simulink model "quadcopter_model_MAIN"  (R2022b)
settings: Solver=FixedStepAuto  StartTime=0.0  StopTime=inf  FixedStep=0.002  RelTol=1e-3
values from neighbouring files (symbols this model uses):
  altToPrsBias = 101270.95    [load_model_parameters.m]
  altToPrsGain = 12.0173    [load_model_parameters.m]
  D = zeros(size(C,1), size(B,2))    [integral_state_feedback.m]    (also in output_feedback.m)
  inverse_mixer_matrix = [1  1  1  1 ... (first row only)    [load_model_parameters.m]
  ms2_to_mg = (1/9.80665)*1000    (= 101.971621298)    [load_model_parameters.m]
  ms_to_cms = 100    [load_model_parameters.m]
  SampleTime = 0.002    [load_model_parameters.m]
undefined symbols (not defined in the file or in its folder): Payload
libraries: uavmavlinklib x11, simulink x3, px4MAVLinkBridgelib x2, robotcorelib x2, sharedtransform x1, sensorinslib x1, mspsensorlib x1
settings Model: ExtModeTrigDuration=10  Creator=paolo  LastModifiedBy=paolo

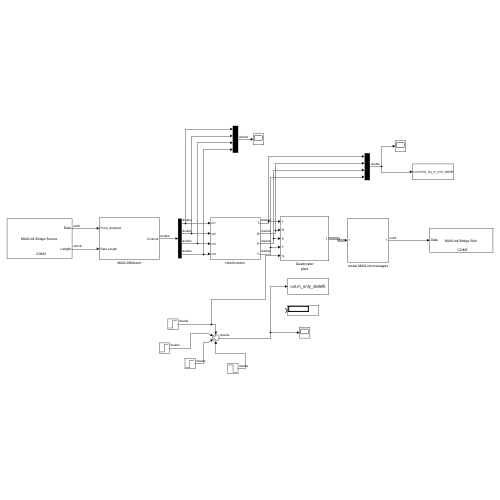
[thumbnail: Simulink's stored preview of the top-level diagram]
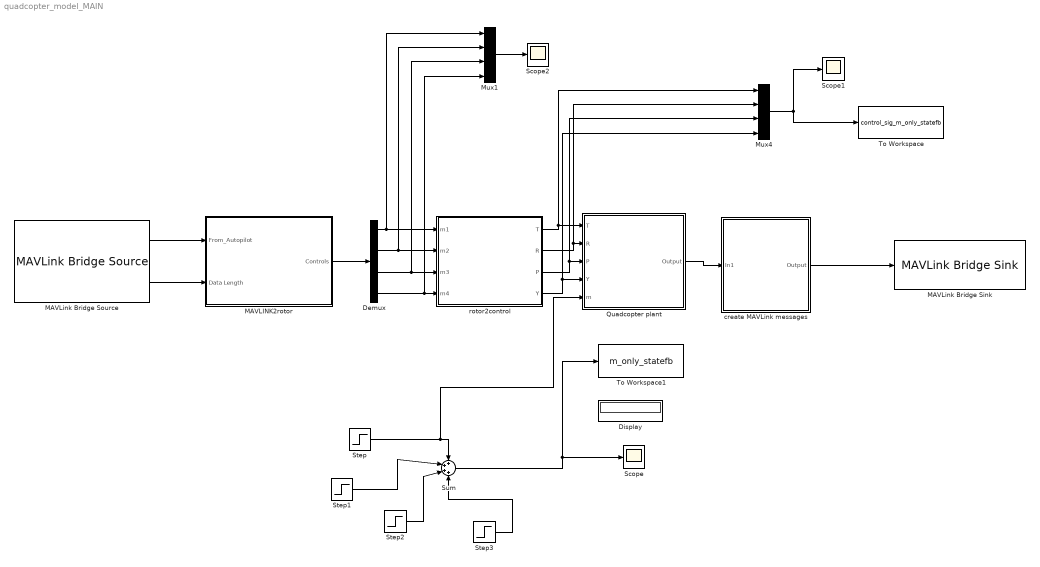
== system quadcopter_model_MAIN ==
  Demux : Demux
  Display : Display
  MAVLINK2rotor : Subsystem
  MAVLink Bridge Sink : px4MAVLinkBridgelib/MAVLink Bridge Sink  PixhawkSerialPorttemp=Specify manually  PixhawkSerialPortManually=COM3  FieldTable={ 'UDP', '127.0.0.1', '14550' }
  MAVLink Bridge Source : px4MAVLinkBridgelib/MAVLink Bridge Source  PixhawkSerialPorttemp=Specify manually  PixhawkSerialPortManually=COM3  dataLength=1024  FieldTable={ 'UDP', '127.0.0.1', '14550' }  SampleTime=SampleTime
  Mux1 : Mux
  Mux4 : Mux
  Quadcopter plant : Subsystem
  Scope : Scope
  Scope1 : Scope
  Scope2 : Scope
  Step : Step  Time=0  After=1.2  SampleTime=0
  Step1 : Step  Time=20  After=1.2  SampleTime=0
  Step2 : Step  Time=40  After=1.2  SampleTime=0
  Step3 : Step  Time=70  After=-2.4  SampleTime=0
  Sum : Sum  Inputs=++++
  To Workspace : ToWorkspace  VariableName=control_sig_m_only_statefb  SampleTime=-1
  To Workspace1 : ToWorkspace  VariableName=m_only_statefb  SampleTime=-1
  create MAVLink messages : Subsystem
  "rotor2control " : Subsystem
  wires:
  Demux/2 -> Mux1/2, "rotor2control "/2(m2)
  Demux/1 -> Mux1/1, "rotor2control "/1(m1)
  Demux/3 -> Mux1/3, "rotor2control "/3(m3)
  Demux/4 -> Mux1/4, "rotor2control "/4(m4)
  Quadcopter plant/1(Output) -> create MAVLink messages/1(In1)
  MAVLink Bridge Source/1 -> MAVLINK2rotor/1(From_Autopilot)
  MAVLink Bridge Source/2 -> MAVLINK2rotor/2(Data Length)
  MAVLINK2rotor/1(Controls) -> Demux/1
  "rotor2control "/3(P) -> Mux4/3, Quadcopter plant/3(P)
  "rotor2control "/4(Y) -> Mux4/4, Quadcopter plant/4(Y)
  "rotor2control "/1(T) -> Mux4/1, Quadcopter plant/1(T)
  "rotor2control "/2(R) -> Mux4/2, Quadcopter plant/2(R)
  Mux4/1 -> To Workspace/1, Scope1/1
  Mux1/1 -> Scope2/1
  Sum/1 -> To Workspace1/1, Scope/1
  Step/1 -> Quadcopter plant/5(m), Sum/1
  Step1/1 -> Sum/2
  Step2/1 -> Sum/3
  Step3/1 -> Sum/4
  create MAVLink messages/1(Output) -> MAVLink Bridge Sink/1

== system quadcopter_model_MAIN/MAVLINK2rotor ==
  From_Autopilot : Inport
  Data Length : Inport  Port=2
  Enabled Subsystem1 : Subsystem  TreatAsAtomicUnit=on
  "Input Signal " : Subsystem
  Controls : Outport
  wires:
  Enabled Subsystem1/1(Controls) -> Controls/1
  Data Length/1 -> "Input Signal "/2(Data Length)
  "Input Signal "/1(Signal) -> Enabled Subsystem1/1(byteStreamInput)
  From_Autopilot/1 -> "Input Signal "/1(From_Autopilot)

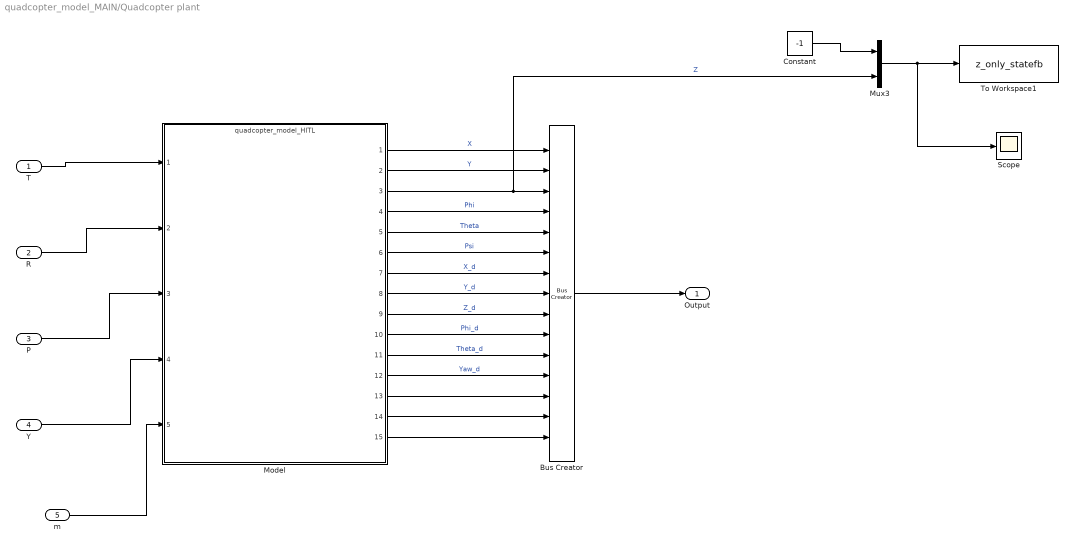
== system quadcopter_model_MAIN/Quadcopter plant ==
  T : Inport
  R : Inport  Port=2
  P : Inport  Port=3
  Y : Inport  Port=4
  m : Inport  Port=5
  Bus Creator : BusCreator  Inputs=15
  Constant : Constant  Value=-1
  Model : ModelReference  ModelNameDialog=quadcopter_model_HITL.slx  SimulationMode=Normal  ModelReferenceVersion=1.131
  Mux3 : Mux  Inputs=2
  Scope : Scope
  To Workspace1 : ToWorkspace  VariableName=z_only_statefb  SampleTime=-1
  Output : Outport
  wires:
  Bus Creator/1 -> Output/1
  R/1 -> Model/2
  T/1 -> Model/1
  P/1 -> Model/3
  Y/1 -> Model/4
  Model/1 -> Bus Creator/1  "X"
  Model/2 -> Bus Creator/2  "Y"
  Model/3 -> Mux3/2, Bus Creator/3  "Z"
  Model/4 -> Bus Creator/4  "Phi"
  Model/5 -> Bus Creator/5  "Theta"
  Model/6 -> Bus Creator/6  "Psi"
  Model/7 -> Bus Creator/7  "X_d"
  Model/8 -> Bus Creator/8  "Y_d"
  Model/9 -> Bus Creator/9  "Z_d"
  Model/10 -> Bus Creator/10  "Phi_d"
  Model/11 -> Bus Creator/11  "Theta_d"
  Model/12 -> Bus Creator/12  "Yaw_d"
  Model/13 -> Bus Creator/13
  Model/14 -> Bus Creator/14
  Model/15 -> Bus Creator/15
  Mux3/1 -> Scope/1, To Workspace1/1
  m/1 -> Model/5
  Constant/1 -> Mux3/1

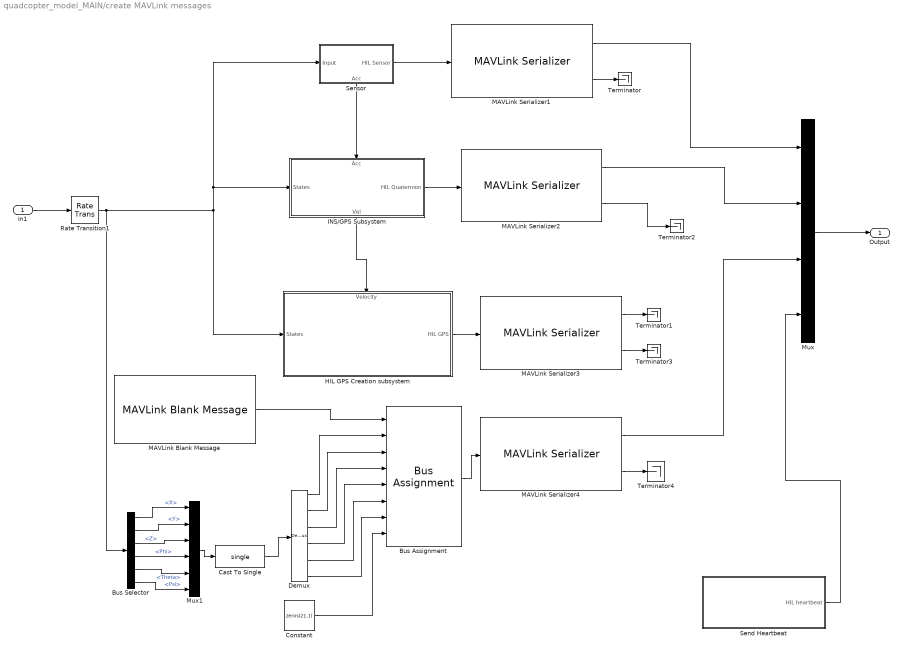
== system quadcopter_model_MAIN/create MAVLink messages ==
  In1 : Inport
  Bus Assignment : BusAssignment  AssignedSignals=Payload.x,Payload.y,Payload.z,Payload.roll,Payload.pitch,Payload.yaw,Payload.covariance
  Bus Selector : BusSelector  OutputSignals=X,Y,Z,Phi,Theta,Psi
  Cast To Single : DataTypeConversion  OutDataTypeStr=single  SaturateOnIntegerOverflow=off  RndMeth=Floor
  Constant : Constant  Value=zeros(21,1)  OutDataTypeStr=single
  Demux : Demux  Outputs=6
  HIL GPS Creation subsystem : Subsystem
      settings: PortSchema="{\"entries\":[{\"content\":{\"sides\":[{\"content\":{\"connectorIds\":[\"In1\"]},\"type\":\"ConnectorPlacement.EquallySpacedRectSide\",\"uuid\":\"f4444677-f205-4bd8-9e95-5e6060697dc4\"},{\"content\":{\"connectorIds\":[\"Out1\"],\"side\":\"RIGHT\"},\"type\":\"ConnectorPlacement.EquallySpacedRectSide\",\"uuid\":\"c948a3e0-826b-4d7b-9e4f-6e3881854d5a\"},{\"content\":{\"connectorIds\":[\"In2\"],\"side\":\"TOP\"},\"type\":\"ConnectorPlacement.EquallySpacedRectSide\",\"uuid\":\"82cf0daf-0b59-4b3c-ab0e-258a514f37ad\"},{\"content\":{\"connectorIds\":[],\"side\":\"HIDDEN\"},\"type\":\"ConnectorPlacement.EquallySpacedRectSide\",\"uuid\":\"a794f320-9150-4c05-acf0-96079b0d3066\"}]},\"type\":\"ConnectorPlacement.EquallySpacedConnector\",\"uuid\":\"8d0915ff-9064-46da-be4f-31886e994f25\"}],\"packageUris\":[\"http://schema.mathworks.com/mf0/Connector/R2020b\"],\"version\":\"1.0\"}"
  INS/GPS Subsystem : Subsystem
      settings: PortSchema="{\"entries\":[{\"content\":{\"sides\":[{\"content\":{\"connectorIds\":[\"In1\"]},\"type\":\"ConnectorPlacement.EquallySpacedRectSide\",\"uuid\":\"bd7d303d-974a-4dd9-8d27-04cf87176bd7\"},{\"content\":{\"connectorIds\":[\"Out1\"],\"side\":\"RIGHT\"},\"type\":\"ConnectorPlacement.EquallySpacedRectSide\",\"uuid\":\"9b60b4cf-af27-4ca7-86b7-e75d27668f15\"},{\"content\":{\"connectorIds\":[\"In2\"],\"side\":\"TOP\"},\"type\":\"ConnectorPlacement.EquallySpacedRectSide\",\"uuid\":\"cd4d20a6-3033-4c65-942d-f02a7fa933e8\"},{\"content\":{\"connectorIds\":[\"Out2\"],\"side\":\"BOTTOM\"},\"type\":\"ConnectorPlacement.EquallySpacedRectSide\",\"uuid\":\"d837ff15-3ee7-4ba9-aab0-0378a7633b3a\"},{\"content\":{\"connectorIds\":[],\"side\":\"HIDDEN\"},\"type\":\"ConnectorPlacement.EquallySpacedRectSide\",\"uuid\":\"eefe2c49-f98f-4c11-8e75-b071b558b610\"}]},\"type\":\"ConnectorPlacement.EquallySpacedConnector\",\"uuid\":\"bd9fca06-cb18-49af-bec9-4d4823ab7b04\"}],\"packageUris\":[\"http://schema.mathworks.com/mf0/Connector/R2020b\"],\"version\":\"1.0\"}"
  MAVLink Blank Message : uavmavlinklib/MAVLink Blank Message  dialectSource=Select from standard MAVLink dialects  dialect=common.xml  dialectCustom=common.xml  version=2  messageType=VISION_POSITION_ESTIMATE  SystemID=2  ComponentID=51  SampleTime=SampleTime
  MAVLink Serializer1 : uavmavlinklib/MAVLink Serializer  dialectSource=Select from standard MAVLink dialects  dialect=common.xml  dialectCustom=common.xml  version=2  messageType=HIL_SENSOR
  MAVLink Serializer2 : uavmavlinklib/MAVLink Serializer  dialectSource=Select from standard MAVLink dialects  dialect=common.xml  dialectCustom=common.xml  version=2  messageType=HIL_STATE_QUATERNION
  MAVLink Serializer3 : uavmavlinklib/MAVLink Serializer  dialectSource=Select from standard MAVLink dialects  dialect=common.xml  dialectCustom=common.xml  version=2  messageType=HIL_GPS
  MAVLink Serializer4 : uavmavlinklib/MAVLink Serializer  dialectSource=Select from standard MAVLink dialects  dialect=common.xml  dialectCustom=common.xml  version=2  messageType=VISION_POSITION_ESTIMATE
  Mux : Mux
  Mux1 : Mux  Inputs=6
  Rate Transition1 : RateTransition
  Send Heartbeat : Subsystem
  Sensor : Subsystem
      settings: PortSchema="{\"entries\":[{\"content\":{\"sides\":[{\"content\":{\"connectorIds\":[\"In1\"]},\"type\":\"ConnectorPlacement.EquallySpacedRectSide\",\"uuid\":\"21193992-b942-4f37-96b2-3e2427de7da2\"},{\"content\":{\"connectorIds\":[\"Out1\"],\"side\":\"RIGHT\"},\"type\":\"ConnectorPlacement.EquallySpacedRectSide\",\"uuid\":\"d922d103-9e57-4e28-9b8a-adf9b3c9706e\"},{\"content\":{\"connectorIds\":[],\"side\":\"TOP\"},\"type\":\"ConnectorPlacement.EquallySpacedRectSide\",\"uuid\":\"3a83b87e-a741-40cd-8150-d56bfba02a64\"},{\"content\":{\"connectorIds\":[\"Out2\"],\"side\":\"BOTTOM\"},\"type\":\"ConnectorPlacement.EquallySpacedRectSide\",\"uuid\":\"dc4544bd-54e8-48b3-894a-72b94a1b8319\"}]},\"type\":\"ConnectorPlacement.EquallySpacedConnector\",\"uuid\":\"35070408-6205-47b4-b515-794d29bbd2ff\"}],\"packageUris\":[\"http://schema.mathworks.com/mf0/Connector/R2020b\"],\"version\":\"1.0\"}"
  Terminator{,1..4} (5 alike) : Terminator
  Output : Outport
  wires:
  INS/GPS Subsystem/2(Vel) -> HIL GPS Creation subsystem/2(Velocity)
  Sensor/2(Acc) -> INS/GPS Subsystem/2(Acc)
  Send Heartbeat/1(HIL heartbeat) -> Mux/4
  MAVLink Serializer3/2 -> Terminator3/1
  HIL GPS Creation subsystem/1(HIL GPS) -> MAVLink Serializer3/1
  MAVLink Serializer1/2 -> Terminator/1
  Mux/1 -> Output/1
  MAVLink Serializer1/1 -> Mux/1
  MAVLink Serializer2/2 -> Terminator2/1
  Sensor/1(HIL Sensor) -> MAVLink Serializer1/1
  INS/GPS Subsystem/1(HIL Quaternion) -> MAVLink Serializer2/1
  Rate Transition1/1 -> Sensor/1(Input), INS/GPS Subsystem/1(States), HIL GPS Creation subsystem/1(States), Bus Selector/1
  In1/1 -> Rate Transition1/1
  MAVLink Serializer3/1 -> Terminator1/1
  Bus Assignment/1 -> MAVLink Serializer4/1
  MAVLink Blank Message/1 -> Bus Assignment/1
  MAVLink Serializer4/2 -> Terminator4/1
  MAVLink Serializer4/1 -> Mux/3
  Constant/1 -> Bus Assignment/8
  Bus Selector/4 -> Mux1/4  "<Phi>"
  Bus Selector/3 -> Mux1/3  "<Z>"
  Bus Selector/5 -> Mux1/5  "<Theta>"
  Bus Selector/2 -> Mux1/2  "<Y>"
  Bus Selector/6 -> Mux1/6  "<Psi>"
  Bus Selector/1 -> Mux1/1  "<X>"
  Mux1/1 -> Cast To Single/1
  Cast To Single/1 -> Demux/1
  Demux/1 -> Bus Assignment/2
  Demux/2 -> Bus Assignment/3
  Demux/3 -> Bus Assignment/4
  Demux/4 -> Bus Assignment/5
  Demux/5 -> Bus Assignment/6
  Demux/6 -> Bus Assignment/7
  MAVLink Serializer2/1 -> Mux/2

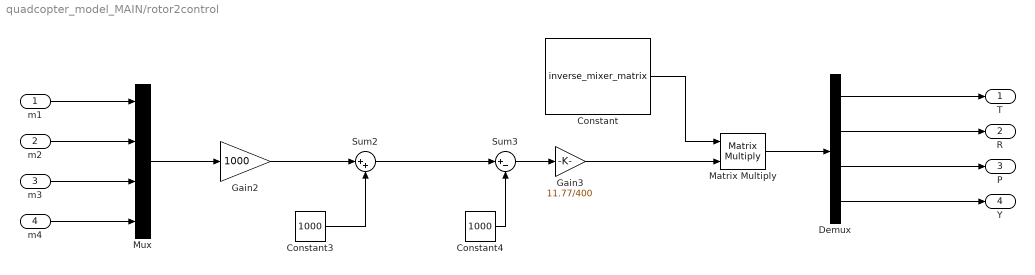
== system quadcopter_model_MAIN/rotor2control  ==
  m1 : Inport
  m2 : Inport  Port=2
  m3 : Inport  Port=3
  m4 : Inport  Port=4
  Constant : Constant  Value=inverse_mixer_matrix
  Constant3 : Constant  Value=1000
  Constant4 : Constant  Value=1000
  Demux : Demux
  Gain2 : Gain  Gain=1000
  Gain3 : Gain  Gain=11.77/400
  Matrix Multiply : Product  Multiplication=Matrix(*)
  Mux : Mux
  Sum2 : Sum  Inputs=|++
  Sum3 : Sum  Inputs=|+-
  T : Outport
  R : Outport  Port=2
  P : Outport  Port=3
  Y : Outport  Port=4
  wires:
  m1/1 -> Mux/1
  m2/1 -> Mux/2
  m3/1 -> Mux/3
  m4/1 -> Mux/4
  Constant/1 -> Matrix Multiply/1
  Matrix Multiply/1 -> Demux/1
  Demux/1 -> T/1
  Demux/2 -> R/1
  Demux/3 -> P/1
  Demux/4 -> Y/1
  Sum3/1 -> Gain3/1
  Constant4/1 -> Sum3/2
  Sum2/1 -> Sum3/1
  Constant3/1 -> Sum2/2
  Gain2/1 -> Sum2/1
  Mux/1 -> Gain2/1
  Gain3/1 -> Matrix Multiply/2

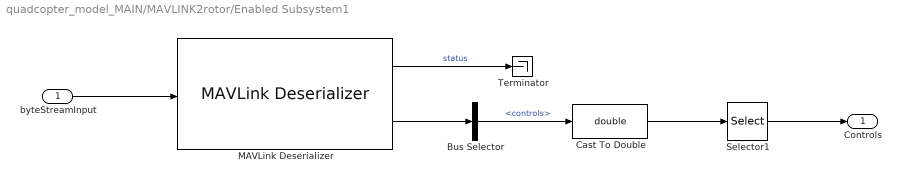
== system quadcopter_model_MAIN/MAVLINK2rotor/Enabled Subsystem1 ==
  byteStreamInput : Inport
  Bus Selector : BusSelector  OutputSignals=Payload.controls
  Cast To Double : DataTypeConversion  OutDataTypeStr=double  SaturateOnIntegerOverflow=off  RndMeth=Floor
  MAVLink Deserializer : uavmavlinklib/MAVLink Deserializer  dialectSource=Select from standard MAVLink dialects  dialect=common.xml  dialectCustom=common.xml  version=2  messageType=HIL_ACTUATOR_CONTROLS  inputDataLength=off  SystemIDFilter=off  systemID=1  ComponentIDFilter=off  componentID=1  queueMsg=off  queueMsgSize=50  dropNum=off
  Selector1 : Selector  InputPortWidth=16  IndexOptions=Index vector (dialog)  Indices=[1:4]  OutputSizes=1
  Terminator : Terminator
  Controls : Outport
  wires:
  Selector1/1 -> Controls/1
  MAVLink Deserializer/1 -> Terminator/1  "status"
  Bus Selector/1 -> Cast To Double/1  "<controls>"
  MAVLink Deserializer/2 -> Bus Selector/1
  byteStreamInput/1 -> MAVLink Deserializer/1
  Cast To Double/1 -> Selector1/1

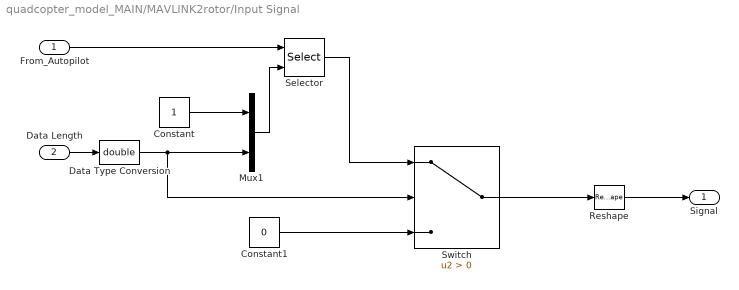
== system quadcopter_model_MAIN/MAVLINK2rotor/Input Signal  ==
  From_Autopilot : Inport
  Data Length : Inport  Port=2
  Constant : Constant
  Constant1 : Constant  Value=0  OutDataTypeStr=uint8  SampleTime=-1
  Data Type Conversion : DataTypeConversion  OutDataTypeStr=double  SaturateOnIntegerOverflow=off  RndMeth=Floor
  Mux1 : Mux  Inputs=2
  Reshape : Reshape
  Selector : Selector  InputPortWidth=1024  IndexOptions=Starting and ending indices (port)  Indices=[1 3]  OutputSizes=1
  Switch : Switch  Criteria=u2 > Threshold  SaturateOnIntegerOverflow=off  InputSameDT=off
  Signal : Outport
  wires:
  Reshape/1 -> Signal/1
  Mux1/1 -> Selector/2
  Data Length/1 -> Data Type Conversion/1
  Constant/1 -> Mux1/1
  Selector/1 -> Switch/1
  From_Autopilot/1 -> Selector/1
  Constant1/1 -> Switch/3
  Switch/1 -> Reshape/1
  Data Type Conversion/1 -> Switch/2, Mux1/2

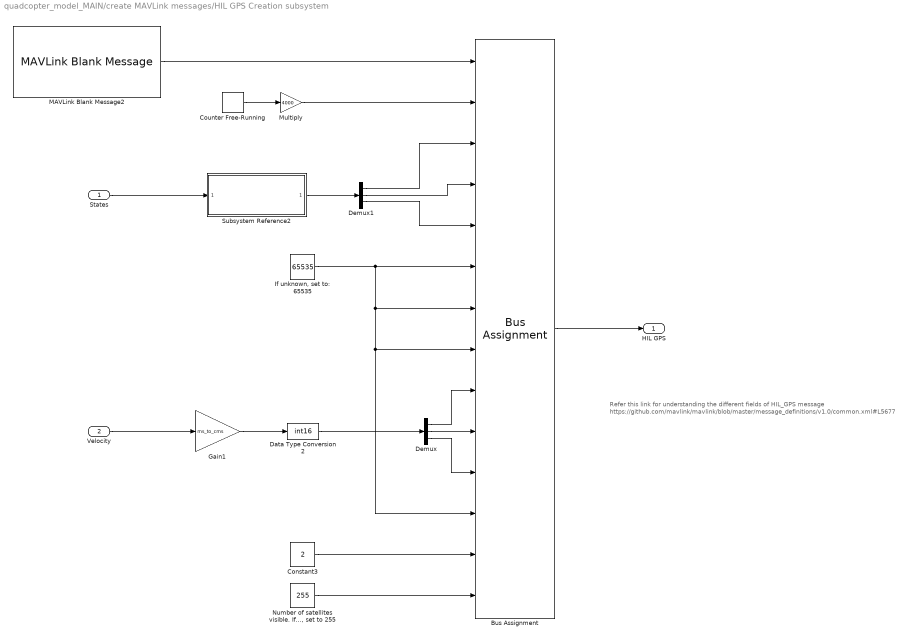
== system quadcopter_model_MAIN/create MAVLink messages/HIL GPS Creation subsystem ==
  note: Refer this link for understanding the different fields of HIL_GPS message https://github.com/mavlink/mavlink/blob/master/message_definitions/v1.0/common.xml#L5677
  States : Inport
  Velocity : Inport  Port=2
  Bus Assignment : BusAssignment  AssignedSignals=Payload.time_usec,Payload.lat,Payload.lon,Payload.alt,Payload.eph,Payload.epv,Payload.vel,Payload.vn,Payload.ve,Payload.vd,Payload.cog,Payload.fix_type,Payload.satellites_visible
  Constant3 : Constant  Value=2  OutDataTypeStr=Inherit: Inherit via back propagation
  Counter Free-Running : simulink/Sources/Counter Free-Running  NumBits=64  tsamp=-1
  Data Type Conversion2 : DataTypeConversion  OutDataTypeStr=int16  SaturateOnIntegerOverflow=off  RndMeth=Floor
  Demux : Demux  Outputs=3
  Demux1 : Demux  Outputs=3
  Gain1 : Gain  Gain=ms_to_cms
  "If unknown, set to: 65535" : Constant  Value=65535  OutDataTypeStr=Inherit: Inherit via back propagation
  MAVLink Blank Message2 : uavmavlinklib/MAVLink Blank Message  dialectSource=Select from standard MAVLink dialects  dialect=common.xml  dialectCustom=common.xml  version=2  messageType=HIL_GPS  SystemID=2  ComponentID=51  SampleTime=SampleTime
  Multiply : Gain  Gain=4000  OutDataTypeStr=Inherit: Inherit via back propagation
  "Number of satellites visible. If unknown, set to 255" : Constant  Value=255  OutDataTypeStr=Inherit: Inherit via back propagation
  Subsystem Reference2 : Subsystem  ReferencedSubsystem=Create_LLA_from_States
  HIL GPS : Outport
  wires:
  MAVLink Blank Message2/1 -> Bus Assignment/1
  Counter Free-Running/1 -> Multiply/1
  Multiply/1 -> Bus Assignment/2
  Bus Assignment/1 -> HIL GPS/1
  "Number of satellites visible. If unknown, set to 255"/1 -> Bus Assignment/14
  "If unknown, set to: 65535"/1 -> Bus Assignment/12, Bus Assignment/8, Bus Assignment/7, Bus Assignment/6
  Constant3/1 -> Bus Assignment/13
  Gain1/1 -> Data Type Conversion2/1
  Velocity/1 -> Gain1/1
  Data Type Conversion2/1 -> Demux/1
  Demux/2 -> Bus Assignment/10
  Demux/1 -> Bus Assignment/9
  Demux/3 -> Bus Assignment/11
  States/1 -> Subsystem Reference2/1
  Subsystem Reference2/1 -> Demux1/1
  Demux1/1 -> Bus Assignment/3
  Demux1/2 -> Bus Assignment/4
  Demux1/3 -> Bus Assignment/5

== system quadcopter_model_MAIN/create MAVLink messages/INS//GPS Subsystem ==
  States : Inport
  Acc : Inport  Port=2
  HIL Quaternion Creation Subsystem : Subsystem
  INS : Subsystem
  HIL Quaternion : Outport
  Vel : Outport  Port=2
  wires:
  HIL Quaternion Creation Subsystem/1(HIL Quaternion) -> HIL Quaternion/1
  States/1 -> HIL Quaternion Creation Subsystem/2(States), INS/1(States)
  Acc/1 -> HIL Quaternion Creation Subsystem/1(Acc)
  INS/1(Vel) -> Vel/1

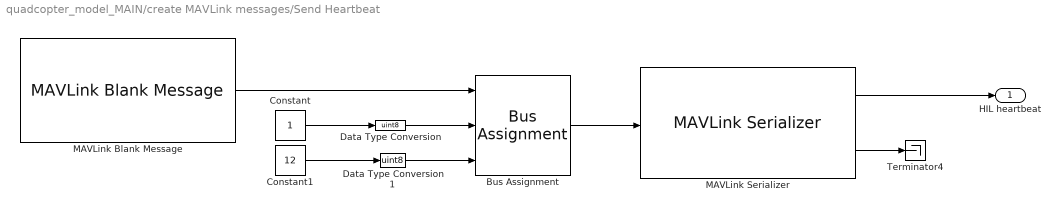
== system quadcopter_model_MAIN/create MAVLink messages/Send Heartbeat ==
  Bus Assignment : BusAssignment  AssignedSignals=Payload.autopilot,Payload.type
  Constant : Constant  SampleTime=SampleTime
  Constant1 : Constant  Value=12  SampleTime=SampleTime
  Data Type Conversion : DataTypeConversion  OutDataTypeStr=uint8  SaturateOnIntegerOverflow=off  RndMeth=Floor
  Data Type Conversion1 : DataTypeConversion  OutDataTypeStr=uint8  SaturateOnIntegerOverflow=off  RndMeth=Floor
  MAVLink Blank Message : uavmavlinklib/MAVLink Blank Message  dialectSource=Select from standard MAVLink dialects  dialect=common.xml  dialectCustom=common.xml  version=2  messageType=HEARTBEAT  SystemID=2  ComponentID=51  SampleTime=SampleTime
  MAVLink Serializer : uavmavlinklib/MAVLink Serializer  dialectSource=Select from standard MAVLink dialects  dialect=common.xml  dialectCustom=common.xml  version=2  messageType=HEARTBEAT
  Terminator4 : Terminator
  HIL heartbeat : Outport
  wires:
  Bus Assignment/1 -> MAVLink Serializer/1
  Constant/1 -> Data Type Conversion/1
  MAVLink Serializer/1 -> HIL heartbeat/1
  Data Type Conversion1/1 -> Bus Assignment/3
  Data Type Conversion/1 -> Bus Assignment/2
  MAVLink Serializer/2 -> Terminator4/1
  Constant1/1 -> Data Type Conversion1/1
  MAVLink Blank Message/1 -> Bus Assignment/1

== system quadcopter_model_MAIN/create MAVLink messages/Sensor ==
  Input : Inport
  Hil Sensor Creation subsystem : Subsystem
  IMU Subsystem : Subsystem
  HIL Sensor : Outport
  Acc : Outport  Port=2
  wires:
  Input/1 -> Hil Sensor Creation subsystem/4(States), IMU Subsystem/1(States)
  IMU Subsystem/1(Acc) -> Acc/1, Hil Sensor Creation subsystem/1(Acc)
  IMU Subsystem/2(Gyro) -> Hil Sensor Creation subsystem/2(Gyro)
  IMU Subsystem/3(Mag) -> Hil Sensor Creation subsystem/3(Mag)
  Hil Sensor Creation subsystem/1(HIL Sensor) -> HIL Sensor/1

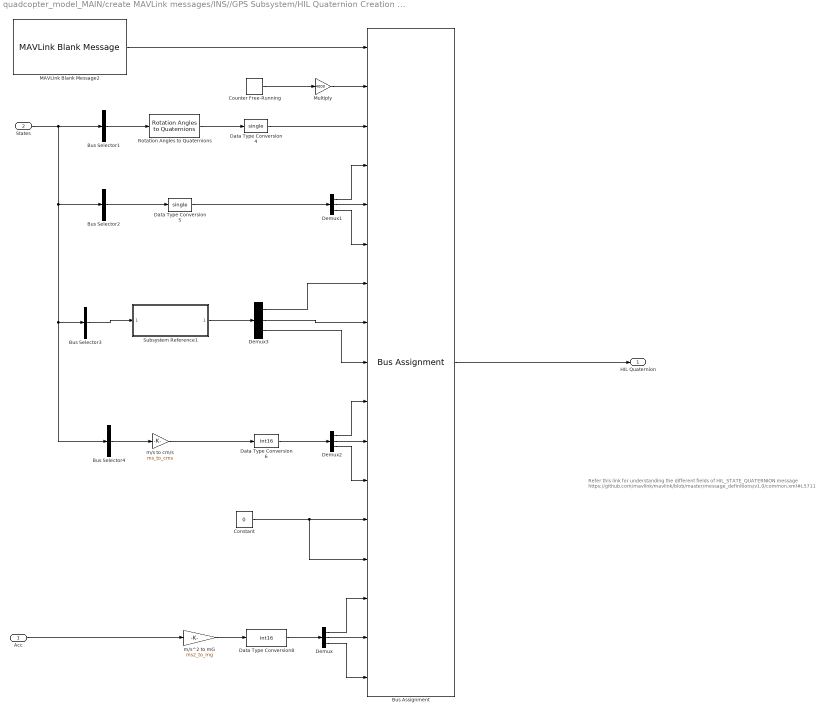
== system quadcopter_model_MAIN/create MAVLink messages/INS//GPS Subsystem/HIL Quaternion Creation Subsystem ==
  note: Refer this link for understanding the different fields of HIL_STATE_QUATERNION message https://github.com/mavlink/mavlink/blob/master/message_definitions/v1.0/common.xml#L5711
  Acc : Inport
  States : Inport  Port=2
  Bus Assignment : BusAssignment  AssignedSignals=Payload.time_usec,Payload.attitude_quaternion,Payload.rollspeed,Payload.pitchspeed,Payload.yawspeed,Payload.lat,Payload.lon,Payload.alt,Payload.vx,Payload.vy,Payload.vz,Payload.ind_airspeed,Payload.true_airspeed,Payload.xacc,Payload.yacc,Payload.zacc
  Bus Selector1 : BusSelector  OutputSignals=Psi,Theta,Phi  OutputAsBus=on
  Bus Selector2 : BusSelector  OutputSignals=Phi_d,Theta_d,Yaw_d  OutputAsBus=on
  Bus Selector3 : BusSelector  OutputSignals=X,Y,Z  OutputAsBus=on
  Bus Selector4 : BusSelector  OutputSignals=X_d,Y_d,Z_d  OutputAsBus=on
  Constant : Constant  Value=0  OutDataTypeStr=Inherit: Inherit via back propagation
  Counter Free-Running : simulink/Sources/Counter Free-Running  NumBits=64  tsamp=-1
  Data Type Conversion4 : DataTypeConversion  OutDataTypeStr=single  SaturateOnIntegerOverflow=off  RndMeth=Floor
  Data Type Conversion5 : DataTypeConversion  OutDataTypeStr=single  SaturateOnIntegerOverflow=off  RndMeth=Floor
  Data Type Conversion6 : DataTypeConversion  OutDataTypeStr=int16  SaturateOnIntegerOverflow=off  RndMeth=Floor
  Data Type Conversion8 : DataTypeConversion  OutDataTypeStr=int16  SaturateOnIntegerOverflow=off  RndMeth=Floor
  Demux{,1..3} (4 alike) : Demux  Outputs=3
  MAVLink Blank Message2 : uavmavlinklib/MAVLink Blank Message  dialectSource=Select from standard MAVLink dialects  dialect=common.xml  dialectCustom=common.xml  version=2  messageType=HIL_STATE_QUATERNION  SystemID=2  ComponentID=51  SampleTime=SampleTime
  Multiply : Gain  Gain=4000  OutDataTypeStr=Inherit: Inherit via back propagation
  Rotation Angles to Quaternions : sharedtransform/Rotation Angles to Quaternions  rotationOrder=ZYX  aMode=aMode
  Subsystem Reference1 : Subsystem  ReferencedSubsystem=Create_LLA_from_States
  m/s to cm/s : Gain  Gain=ms_to_cms
  m/s^2 to mG : Gain  Gain=ms2_to_mg
  HIL Quaternion : Outport
  wires:
  Counter Free-Running/1 -> Multiply/1
  MAVLink Blank Message2/1 -> Bus Assignment/1
  Multiply/1 -> Bus Assignment/2
  Bus Assignment/1 -> HIL Quaternion/1
  States/1 -> Bus Selector1/1, Bus Selector2/1, Bus Selector4/1, Bus Selector3/1
  Rotation Angles to Quaternions/1 -> Data Type Conversion4/1
  Data Type Conversion4/1 -> Bus Assignment/3
  Demux/3 -> Bus Assignment/17
  Demux/1 -> Bus Assignment/15
  Demux/2 -> Bus Assignment/16
  Constant/1 -> Bus Assignment/14, Bus Assignment/13
  m/s to cm/s/1 -> Data Type Conversion6/1
  Data Type Conversion6/1 -> Demux2/1
  Demux2/3 -> Bus Assignment/12
  Demux2/2 -> Bus Assignment/11
  Demux2/1 -> Bus Assignment/10
  Data Type Conversion8/1 -> Demux/1
  Acc/1 -> m/s^2 to mG/1
  m/s^2 to mG/1 -> Data Type Conversion8/1
  Bus Selector1/1 -> Rotation Angles to Quaternions/1
  Data Type Conversion5/1 -> Demux1/1
  Demux1/3 -> Bus Assignment/6
  Demux1/2 -> Bus Assignment/5
  Demux1/1 -> Bus Assignment/4
  Bus Selector2/1 -> Data Type Conversion5/1
  Bus Selector3/1 -> Subsystem Reference1/1
  Bus Selector4/1 -> m/s to cm/s/1
  Subsystem Reference1/1 -> Demux3/1
  Demux3/1 -> Bus Assignment/7
  Demux3/2 -> Bus Assignment/8
  Demux3/3 -> Bus Assignment/9

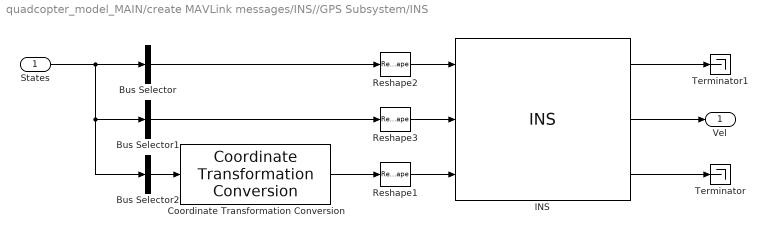
== system quadcopter_model_MAIN/create MAVLink messages/INS//GPS Subsystem/INS ==
  States : Inport
  Bus Selector : BusSelector  OutputSignals=X,Y,Z  OutputAsBus=on
  Bus Selector1 : BusSelector  OutputSignals=X_d,Y_d,Z_d  OutputAsBus=on
  Bus Selector2 : BusSelector  OutputSignals=Psi,Theta,Phi  OutputAsBus=on
  Coordinate Transformation Conversion : robotcorelib/Coordinate Transformation Conversion  InputRepresentation=Euler Angles  InputEulerSequence=ZYX  ShowTrVecInputPort=on  OutputRepresentation=Quaternion  OutputEulerSequence=ZYX  ShowTrVecOutputPort=on  SimulateUsing=Interpreted execution
  INS : sensorinslib/INS  MountingLocation=[0 0 0]  RollAccuracy=0.2  PitchAccuracy=0.2  YawAccuracy=1  PositionAccuracy=1  VelocityAccuracy=0.05  UseAccelAndAngVel=off  AccelerationAccuracy=0  AngularVelocityAccuracy=0  TimeInput=off  PositionErrorFactor=[0 0 0]  SeedDouble=67  SimulateUsing=Interpreted execution
  Reshape1 : Reshape  OutputDimensionality=Row vector (2-D)
  Reshape2 : Reshape  OutputDimensionality=Row vector (2-D)
  Reshape3 : Reshape  OutputDimensionality=Row vector (2-D)
  Terminator : Terminator
  Terminator1 : Terminator
  Vel : Outport
  wires:
  Bus Selector1/1 -> Reshape3/1
  Bus Selector/1 -> Reshape2/1
  Reshape2/1 -> INS/1
  Bus Selector2/1 -> Coordinate Transformation Conversion/1
  Reshape3/1 -> INS/2
  States/1 -> Bus Selector2/1, Bus Selector1/1, Bus Selector/1
  Coordinate Transformation Conversion/1 -> Reshape1/1
  INS/1 -> Terminator1/1
  INS/3 -> Terminator/1
  INS/2 -> Vel/1
  Reshape1/1 -> INS/3

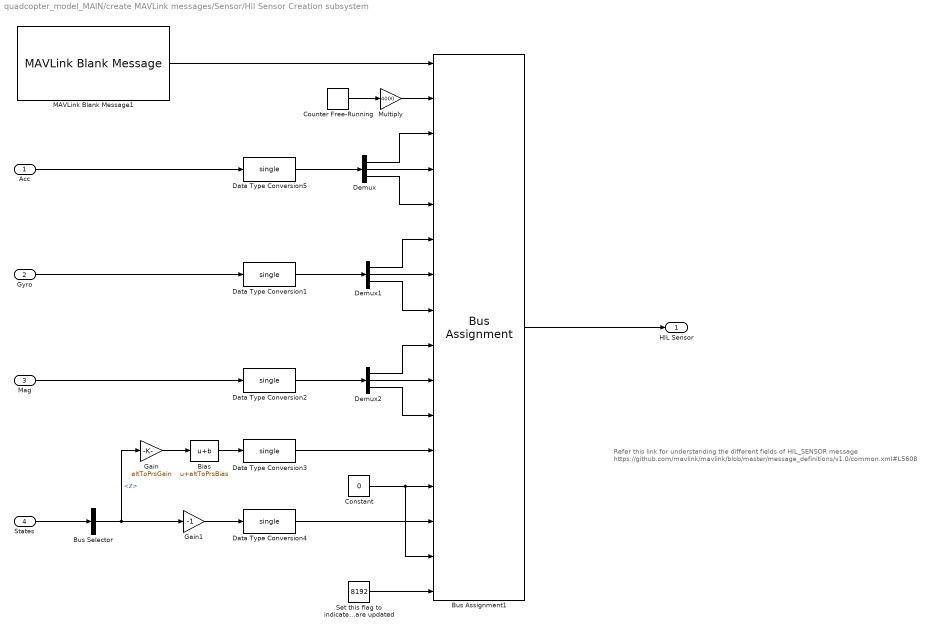
== system quadcopter_model_MAIN/create MAVLink messages/Sensor/Hil Sensor Creation subsystem ==
  note: Refer this link for understanding the different fields of HIL_SENSOR message https://github.com/mavlink/mavlink/blob/master/message_definitions/v1.0/common.xml#L5608
  Acc : Inport
  Gyro : Inport  Port=2
  Mag : Inport  Port=3
  States : Inport  Port=4
  Bias : Bias  Bias=altToPrsBias  SaturateOnIntegerOverflow=off
  Bus Assignment1 : BusAssignment  AssignedSignals=Payload.time_usec,Payload.xacc,Payload.yacc,Payload.zacc,Payload.xgyro,Payload.ygyro,Payload.zgyro,Payload.xmag,Payload.ymag,Payload.zmag,Payload.abs_pressure,Payload.diff_pressure,Payload.pressure_alt,Payload.temperature,Payload.fields_updated
  Bus Selector : BusSelector  OutputSignals=Z
  Constant : Constant  Value=0  OutDataTypeStr=Inherit: Inherit via back propagation  SampleTime=SampleTime
  Counter Free-Running : simulink/Sources/Counter Free-Running  NumBits=64  tsamp=SampleTime
  Data Type Conversion{1..5} (5 alike) : DataTypeConversion  OutDataTypeStr=single  SaturateOnIntegerOverflow=off  RndMeth=Floor
  Demux : Demux  Outputs=3
  Demux1 : Demux  Outputs=3
  Demux2 : Demux  Outputs=3
  Gain : Gain  Gain=altToPrsGain
  Gain1 : Gain  Gain=-1
  MAVLink Blank Message1 : uavmavlinklib/MAVLink Blank Message  dialectSource=Select from standard MAVLink dialects  dialect=common.xml  dialectCustom=common.xml  version=2  messageType=HIL_SENSOR  SystemID=2  ComponentID=51  SampleTime=SampleTime
  Multiply : Gain  Gain=4000  OutDataTypeStr=Inherit: Inherit via back propagation
  Set this flag to indicate all flags are updated : Constant  Value=8192  OutDataTypeStr=Inherit: Inherit via back propagation  SampleTime=SampleTime
  HIL Sensor : Outport
  wires:
  Data Type Conversion2/1 -> Demux2/1
  Demux1/1 -> Bus Assignment1/6
  Counter Free-Running/1 -> Multiply/1
  Mag/1 -> Data Type Conversion2/1
  Demux1/3 -> Bus Assignment1/8
  Data Type Conversion1/1 -> Demux1/1
  Gyro/1 -> Data Type Conversion1/1
  Bus Assignment1/1 -> HIL Sensor/1
  Set this flag to indicate all flags are updated/1 -> Bus Assignment1/16
  Demux/3 -> Bus Assignment1/5
  Demux2/2 -> Bus Assignment1/10
  Demux2/3 -> Bus Assignment1/11
  Data Type Conversion5/1 -> Demux/1
  Demux/1 -> Bus Assignment1/3
  Multiply/1 -> Bus Assignment1/2
  Constant/1 -> Bus Assignment1/15, Bus Assignment1/13
  MAVLink Blank Message1/1 -> Bus Assignment1/1
  Demux2/1 -> Bus Assignment1/9
  Demux/2 -> Bus Assignment1/4
  Demux1/2 -> Bus Assignment1/7
  Bus Selector/1 -> Gain/1, Gain1/1  "<Z>"
  Acc/1 -> Data Type Conversion5/1
  States/1 -> Bus Selector/1
  Bias/1 -> Data Type Conversion3/1
  Gain/1 -> Bias/1
  Data Type Conversion4/1 -> Bus Assignment1/14
  Data Type Conversion3/1 -> Bus Assignment1/12
  Gain1/1 -> Data Type Conversion4/1

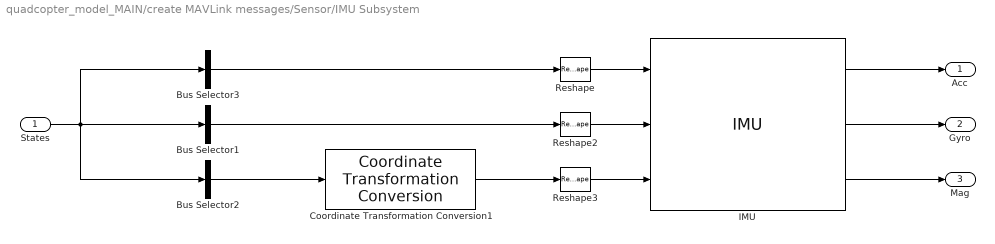
== system quadcopter_model_MAIN/create MAVLink messages/Sensor/IMU Subsystem ==
  States : Inport
  Bus Selector1 : BusSelector  OutputSignals=Phi_d,Theta_d,Yaw_d  OutputAsBus=on
  Bus Selector2 : BusSelector  OutputSignals=Psi,Theta,Phi  OutputAsBus=on
  Bus Selector3 : BusSelector  OutputSignals=x_dd,y_dd,z_dd  OutputAsBus=on
  Coordinate Transformation Conversion1 : robotcorelib/Coordinate Transformation Conversion  InputRepresentation=Euler Angles  InputEulerSequence=ZYX  ShowTrVecInputPort=on  OutputRepresentation=Quaternion  OutputEulerSequence=ZYX  ShowTrVecOutputPort=on  SimulateUsing=Interpreted execution
  IMU : mspsensorlib/IMU  DispRefFrame=NED  Temperature=25  MagneticFieldNED=[ 27.5550, -2.4169, -16.0849 ]  MagneticFieldENU=[ -2.4169, 27.5550, 16.0849 ]  SeedDouble=67  SimulateUsing=Interpreted execution  AccelParamsMeasurementRange=Inf  AccelParamsResolution=0  AccelParamsConstantBias=[ 0, 0, 0 ]  AccelParamsAxesMisalignment=[ 0, 0, 0 ]  AccelParamsNoiseDensity=[ 0, 0, 0 ]  AccelParamsBiasInstability=[ 0, 0, 0 ]  AccelParamsRandomWalk=[ 0, 0, 0 ]  AccelParamsTemperatureBias=[ 0, 0, 0 ]  AccelParamsTemperatureScaleFactor=[ 0, 0, 0 ]  GyroParamsMeasurementRange=Inf  GyroParamsResolution=0  GyroParamsConstantBias=[ 0, 0, 0 ]  GyroParamsAxesMisalignment=[ 0, 0, 0 ]  GyroParamsAccelerationBias=[ 0, 0, 0 ]  GyroParamsNoiseDensity=[ 0, 0, 0 ]  GyroParamsBiasInstability=[ 0, 0, 0 ]  GyroParamsRandomWalk=[ 0, 0, 0 ]  GyroParamsTemperatureBias=[ 0, 0, 0 ]  GyroParamsTemperatureScaleFactor=[ 0, 0, 0 ]  MagParamsMeasurementRange=Inf  MagParamsResolution=0  MagParamsConstantBias=[ 0, 0, 0 ]  MagParamsAxesMisalignment=[ 0, 0, 0 ]  MagParamsNoiseDensity=[ 0, 0, 0 ]  MagParamsBiasInstability=[ 0, 0, 0 ]  MagParamsRandomWalk=[ 0, 0, 0 ]  MagParamsTemperatureBias=[ 0, 0, 0 ]  MagParamsTemperatureScaleFactor=[ 0, 0, 0 ]
  Reshape : Reshape  OutputDimensionality=Row vector (2-D)
  Reshape2 : Reshape  OutputDimensionality=Row vector (2-D)
  Reshape3 : Reshape  OutputDimensionality=Row vector (2-D)
  Acc : Outport
  Gyro : Outport  Port=2
  Mag : Outport  Port=3
  wires:
  Bus Selector1/1 -> Reshape2/1
  Bus Selector2/1 -> Coordinate Transformation Conversion1/1
  IMU/3 -> Mag/1
  Reshape2/1 -> IMU/2
  Bus Selector3/1 -> Reshape/1
  Coordinate Transformation Conversion1/1 -> Reshape3/1
  Reshape/1 -> IMU/1
  IMU/2 -> Gyro/1
  Reshape3/1 -> IMU/3
  States/1 -> Bus Selector3/1, Bus Selector2/1, Bus Selector1/1
  IMU/1 -> Acc/1
